simulink model "L1_0"  (Simulink 7.9)
settings: Solver=ode45  StartTime=0.0  StopTime=10.0  RelTol=1e-3
libraries: simulink x1
settings Model: Creator=Павло  LastModifiedBy=Павло

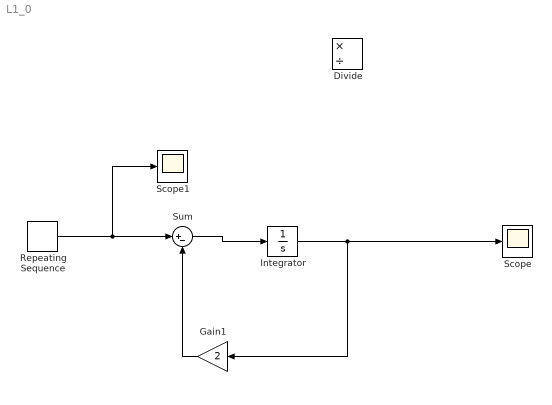
== system L1_0 ==
  Divide : Product  Inputs=*/
  Gain1 : Gain  Gain=2
      settings: AttributesFormatString=2
  Integrator : Integrator
  Repeating Sequence : simulink/Sources/Repeating Sequence  rep_seq_t=[0 2]  rep_seq_y=[1 2]
  Scope : Scope
      settings: TickLabels=on  TimeRange=0.9379378758757522  YMin=0.2922020202020199  YMax=0.54820202020202
  Scope1 : Scope
  Sum : Sum  Inputs=|+-
  wires:
  Repeating Sequence/1 -> Sum/1, Scope1/1
  Gain1/1 -> Sum/2
  Sum/1 -> Integrator/1
  Integrator/1 -> Gain1/1, Scope/1
